simulink library "vehicleLE_cl"  (R2018b)
settings: Solver=VariableStepAuto  StartTime=0.0  StopTime=10.0  RelTol=1e-3
undefined symbols (not defined in the file): dragTurbine, dragTurbine_ul, env, fluidDynamicSurface, fluidDynamicSurface_cl, fuselage, fuselage_cl, surfaceCoefficients, surfaceCoefficients_ul, tethersMoment, tethersMoment_cl, thrAttachPtKinematics, thrAttachPtKinematics_ul, vhcl
libraries: vrlib x7, vectorNormalizer_ul x3, localApparentWind_ul x3, xProdMatrix_ul x2, dynamicPressure_ul x2, dspstat3 x2, dsppolyfun x2, firstOrderFilter_ul x1, simulink x1, alphaBetaLE_ul x1, rotateAboutVec x1, sixDoFDynamics_cl x1
settings Model: Creator=mcobb  LastModifiedBy=jldanie5

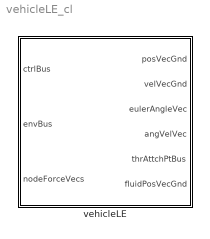
== system vehicleLE_cl ==
  vehicleLE : Subsystem  VariantControl=VSS_vehicle_vehicleLETest  mask{vcl=vhcl, rho=env.water.density.Value, grav=env.gravAccel.Value}
      mask prompts: vcl "Vehicle"; rho "Density"; grav "Gravity"
      mask DialogControl Container9 Prompt: General
      mask DialogControl Container5 Prompt: Vehicle object (OCT.vehicle)
      mask DialogControl ParameterGroupVar Prompt: Environment Object (OCT.env)
      mask Display:
      | image('kite.jpg',[100 100 601 528]/4,'on')
      | 
      | port_label('input',1,'ctrlBus')
      | port_label('input',2,'envBus')
      | port_label('input',3,'nodeForceVecs')
      | 
      | port_label('output',1,'posVecGnd')
      | port_label('output',2,'velVecGnd')
      | port_label('output',3,'eulAng')
      | port_label('output',4,'angVelVec')
      | port_label('output',5,'thrAttchPtBus')
      | port_label('output',6,'fluidPosVecGnd')

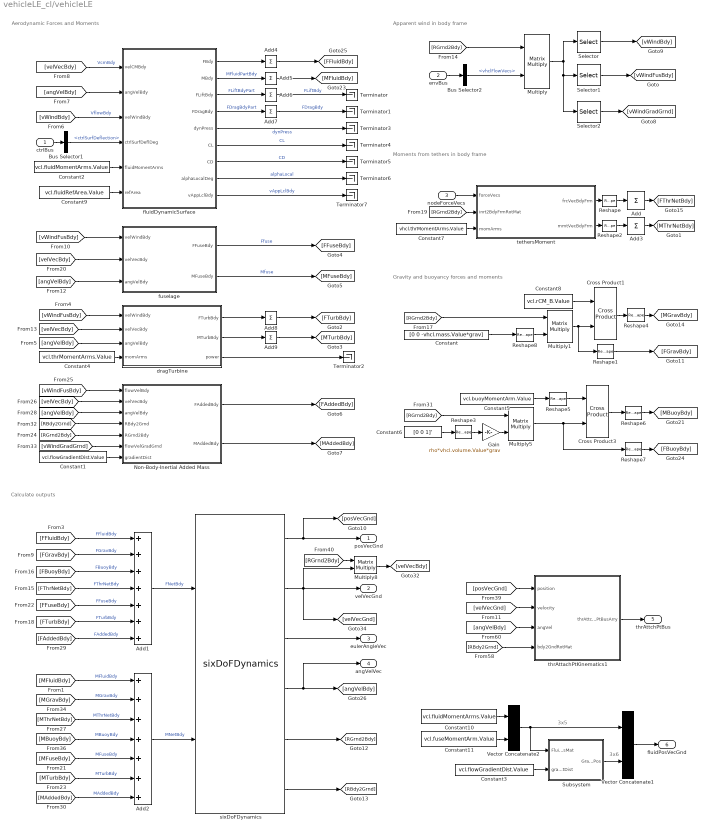
== system vehicleLE_cl/vehicleLE ==
  note: 3x6
  note: 3x5
  note: Calculate outputs
  note: Apparent wind in body frame
  note: Gravity and buoyancy forces and moments
  note: Moments from tethers in body frame
  note: Aerodynamic Forces and Moments
  ctrlBus : Inport  OutDataTypeStr=Bus: fltCtrlBus
  envBus : Inport  Port=2  OutDataTypeStr=Bus: envBus
  nodeForceVecs : Inport  Port=3
  Add : Sum  Inputs=+  CollapseMode=Specified dimension  CollapseDim=2
  Add1 : Sum  Inputs=+++++++
  Add2 : Sum  Inputs=+++++++
  Add3 : Sum  Inputs=+  CollapseMode=Specified dimension  CollapseDim=2
  Add{4..9} (6 alike) : Sum  Inputs=1  CollapseMode=Specified dimension  CollapseDim=2
  Bus Selector1 : BusSelector  OutputSignals=ctrlSurfDeflection
  Bus Selector2 : BusSelector  OutputSignals=vhclFlowVecs
  Constant : Constant  Value=[0 0 -vhcl.mass.Value*grav]
  Constant1 : Constant  Value=vcl.flowGradientDist.Value
  Constant10 : Constant  Value=vcl.fluidMomentArms.Value
  Constant11 : Constant  Value=vcl.fuseMomentArm.Value
  Constant2 : Constant  Value=vcl.fluidMomentArms.Value
  Constant3 : Constant  Value=vcl.flowGradientDist.Value
  Constant4 : Constant  Value=vcl.thrMomentArms.Value  VectorParams1D=off
  Constant5 : Constant  Value=vcl.buoyMomentArm.Value
  Constant6 : Constant  Value=[0 0 1]'
  Constant7 : Constant  Value=vhcl.thrMomentArms.Value
  Constant8 : Constant  Value=vcl.rCM_B.Value
  Constant9 : Constant  Value=vcl.fluidRefArea.Value
  Cross Product1 : vrlib/Utilities/Cross Product
      settings: SourceProductBaseCode=VR
  Cross Product3 : vrlib/Utilities/Cross Product
      settings: SourceProductBaseCode=VR
  Gain : Gain  Gain=rho*vhcl.volume.Value*grav
  Multiply{,1,5,8} (4 alike) : Product  Multiplication=Matrix(*)
  Non-Body-Inertial Added Mass : Subsystem  AncestorBlock=addedMass_cl/Non-Body-Inertial Added Mass  mask{MaMat=vcl.Ma6x6_B.Value}
      mask prompts: MaMat "Added Mass Matrix"
  Reshape : Reshape  OutputDimensionality=Customize  OutputDimensions=[3 vcl.numTethers.Value]
  Reshape{1,3..8} (7 alike) : Reshape  OutputDimensionality=Column vector (2-D)
  Reshape2 : Reshape  OutputDimensionality=Customize  OutputDimensions=[3 vcl.numTethers.Value]
  Selector : Selector  NumberOfDimensions=2  InputPortWidth=3  IndexOptions=Select all,Index vector (dialog)  Indices=[1 3],1:4  OutputSizes=1,1
  Selector1 : Selector  NumberOfDimensions=2  InputPortWidth=3  IndexOptions=Select all,Index vector (dialog)  Indices=[1 3],5  OutputSizes=1,1
  Selector2 : Selector  NumberOfDimensions=2  InputPortWidth=3  IndexOptions=Select all,Index vector (dialog)  Indices=[1 3],6:11  OutputSizes=1,1
  Subsystem : Subsystem
  Terminator{,1..7} (8 alike) : Terminator
  Vector Concatenate1 : Concatenate  Mode=Multidimensional array  ConcatenateDimension=2
  Vector Concatenate2 : Concatenate  Mode=Multidimensional array  ConcatenateDimension=2
  dragTurbine : Subsystem  AncestorBlock=dragTurbine_ul/dragTurbine  TreatAsAtomicUnit=on  mask{rho_fluid=rho, turb_struct=vcl.struct('OCT.turb'), momArms=0}
      mask prompts: rho_fluid "Fluid density"; turb_struct "Turbines structure"; momArms "Turbine Moment Arms"
  fluidDynamicSurface : Subsystem  AncestorBlock=fluidDynamicSurface_cl/fluidDynamicSurface  mask{aeroStruct=vcl.struct('OCT.aeroSurfLE'), fluidDensity=env.water.density.Value}
      mask prompts: aeroStruct "Aerodynamic surface structure"; fluidDensity "Fluid density"
      mask help:
      | Input must be an 1×N struct array with fields:
      |     refArea
      |     aeroCentPosVec
      |     spanUnitVec
      |     chordUnitVec
      |     CL
      |     CD
      |     alpha
      |     GainCL
      |     GainCD
      |
      | where N is the number of aerodynamic surfaces
      settings: MinAlgLoopOccurrences=on
  fuselage : Subsystem  AncestorBlock=fuselage_cl/fuselage  mask{momArm=vcl.fuseMomentArm.Value, fus=vcl.fuse, fusRhoDa=rho}
      mask prompts: momArm "Fuselage Moment Arm"; fus "Fuselage"; fusRhoDa "Density"
      mask DialogControl Container4 Prompt: General
      mask DialogControl Container9 Prompt: Fuselage object (OCT.fuselage)
      mask DialogControl Container8 Prompt: Environment Object (OCT.env)
  sixDoFDynamics : sixDoFDynamics_cl/sixDoFDynamics  vcl=vcl
  tethersMoment : Subsystem  AncestorBlock=tethersMoment_cl/tethersMoment  mask{arms=vcl.struct('OCT.thrAttchLE')}
      mask prompts: arms "Moment arm(s)"
  thrAttachPtKinematics1 : Subsystem  AncestorBlock=thrAttachPtKinematics_ul/thrAttachPtKinematics  InitFcn=thrAttachPtKinematics_init  mask{atchPts=vcl.struct('OCT.thrAttchLE')}
      mask prompts: atchPts "Tether attachment point vec in platform frame"
      mask init:
      | thrAttachPtKinematics_init
  posVecGnd : Outport
  velVecGnd : Outport  Port=2
  eulerAngleVec : Outport  Port=3
  angVelVec : Outport  Port=4
  thrAttchPtBus : Outport  Port=5
  fluidPosVecGnd : Outport  Port=6
  wires:
  sixDoFDynamics/3 -> eulerAngleVec/1
  sixDoFDynamics/1 -> [posVecGnd], posVecGnd/1
  sixDoFDynamics/2 -> Multiply8/2, [velVecGnd], velVecGnd/1
  thrAttachPtKinematics1/1(thrAttchPtBusArry) -> thrAttchPtBus/1
  fluidDynamicSurface/1(FBdy) -> Add4/1
  Constant2/1 -> fluidDynamicSurface/5(fluidMomentArms)
  fluidDynamicSurface/2(MBdy) -> Add5/1  "MFluidPartBdy"
  fluidDynamicSurface/3(FLiftBdy) -> Add6/1  "FLiftBdyPart"
  fluidDynamicSurface/4(FDragBdy) -> Add7/1  "FDragBdyPart"
  fluidDynamicSurface/5(dynPress) -> Terminator3/1  "dynPress"
  fluidDynamicSurface/6(CL) -> Terminator4/1  "CL"
  fluidDynamicSurface/7(CD) -> Terminator5/1  "CD"
  fluidDynamicSurface/8(alphaLocalDeg) -> Terminator6/1  "alphaLocal"
  fluidDynamicSurface/9(vAppLclBdy) -> Terminator7/1  "vAppLclBdy"
  Add4/1 -> [FFluidBdy]
  Add5/1 -> [MFluidBdy]
  Add6/1 -> Terminator/1  "FLiftBdy"
  Add7/1 -> Terminator1/1  "FDragBdy"
  [velVecBdy] -> fluidDynamicSurface/1(velCMBdy)  "VcmBdy"
  [angVelBdy] -> fluidDynamicSurface/2(angVelBdy)
  [vWindBdy] -> fluidDynamicSurface/3(velWindBdy)  "VflowBdy"
  Bus Selector1/1 -> fluidDynamicSurface/4(ctrlSurfDeflDeg)  "<ctrlSurfDeflection>"
  ctrlBus/1 -> Bus Selector1/1
  Constant9/1 -> fluidDynamicSurface/6(refArea)
  [vWindFusBdy] -> fuselage/1(velWindBdy)
  [velVecBdy] -> fuselage/2(velVecBdy)
  [angVelBdy] -> fuselage/3(angVelBdy)
  [vWindFusBdy] -> dragTurbine/1(velWindBdy)
  [velVecBdy] -> dragTurbine/2(velVecBdy)
  [angVelBdy] -> dragTurbine/3(angVelBdy)
  Constant4/1 -> dragTurbine/4(momArms)
  dragTurbine/1(FTurbBdy) -> Add8/1
  dragTurbine/2(MTurbBdy) -> Add9/1
  Add8/1 -> [FTurbBdy]
  Add9/1 -> [MTurbBdy]
  dragTurbine/3(power) -> Terminator2/1
  [vWindFusBdy] -> Non-Body-Inertial Added Mass/1("flowVelBdy ")
  [velVecBdy] -> Non-Body-Inertial Added Mass/2(velVecBdy)
  [angVelBdy] -> Non-Body-Inertial Added Mass/3(angVelBdy)
  [RBdy2Grnd] -> Non-Body-Inertial Added Mass/4(RBdy2Grnd)
  [RGrnd2Bdy] -> Non-Body-Inertial Added Mass/5(RGrnd2Bdy)
  [vWindGradGrnd] -> Non-Body-Inertial Added Mass/6(flowVelGradGrnd)
  Constant1/1 -> Non-Body-Inertial Added Mass/7(gradientDist)
  Non-Body-Inertial Added Mass/1(FAddedBdy) -> [FAddedBdy]
  Constant6/1 -> Reshape3/1
  Reshape3/1 -> Gain/1
  [RGrnd2Bdy] -> Multiply5/1
  Gain/1 -> Multiply5/2
  Constant5/1 -> Reshape5/1
  Reshape5/1 -> Cross Product3/1
  Cross Product3/1 -> Reshape6/1
  Reshape6/1 -> [MBuoyBdy]
  Multiply5/1 -> Reshape7/1, Cross Product3/2
  Reshape7/1 -> [FBuoyBdy]
  Reshape1/1 -> [FGravBdy]
  Multiply1/1 -> Reshape1/1, Cross Product1/2
  fuselage/1(FFuseBdy) -> [FFuseBdy]  "Ffuse"
  fuselage/2(MFuseBdy) -> [MFuseBdy]  "Mfuse"
  Constant/1 -> Reshape8/1
  [RGrnd2Bdy] -> Multiply1/1
  Reshape8/1 -> Multiply1/2
  Constant8/1 -> Cross Product1/1
  Cross Product1/1 -> Reshape4/1
  Reshape4/1 -> [MGravBdy]
  Constant7/1 -> tethersMoment/3(momArms)
  [RGrnd2Bdy] -> tethersMoment/2(inrt2BdyFrmRotMat)
  nodeForceVecs/1 -> tethersMoment/1(forceVecs)
  tethersMoment/1(frcVecBdyFrm) -> Reshape/1
  tethersMoment/2(mmtVecBdyFrm) -> Reshape2/1
  Reshape/1 -> Add/1
  Reshape2/1 -> Add3/1
  Add/1 -> [FThrNetBdy]
  Add3/1 -> [MThrNetBdy]
  [RGrnd2Bdy] -> Multiply/1
  envBus/1 -> Bus Selector2/1
  Bus Selector2/1 -> Multiply/2  "<vhclFlowVecs>"
  Multiply/1 -> Selector/1, Selector2/1, Selector1/1
  Selector/1 -> [vWindBdy]
  Selector1/1 -> [vWindFusBdy]
  Selector2/1 -> [vWindGradGrnd]
  [RGrnd2Bdy] -> Multiply8/1
  Multiply8/1 -> [velVecBdy]
  [FFluidBdy] -> Add1/1  "FFluidBdy"
  [FGravBdy] -> Add1/2  "FGravBdy"
  [FBuoyBdy] -> Add1/3  "FBuoyBdy"
  [FThrNetBdy] -> Add1/4  "FThrNetBdy"
  [FFuseBdy] -> Add1/5  "FFuseBdy"
  [FTurbBdy] -> Add1/6  "FTurbBdy"
  [FAddedBdy] -> Add1/7  "FAddedBdy"
  Add1/1 -> sixDoFDynamics/1  "FNetBdy"
  [MFluidBdy] -> Add2/1  "MFluidBdy"
  [MGravBdy] -> Add2/2  "MGravBdy"
  [MThrNetBdy] -> Add2/3  "MThrNetBdy"
  [MBuoyBdy] -> Add2/4  "MBuoyBdy"
  [MFuseBdy] -> Add2/5  "MFuseBdy"
  [MTurbBdy] -> Add2/6  "MTurbBdy"
  [MAddedBdy] -> Add2/7  "MAddedBdy"
  Add2/1 -> sixDoFDynamics/2  "MNetBdy"
  sixDoFDynamics/5 -> [RGrnd2Bdy]
  sixDoFDynamics/6 -> [RBdy2Grnd]
  [posVecGnd] -> thrAttachPtKinematics1/1(position)
  [velVecGnd] -> thrAttachPtKinematics1/2(velocity)
  [angVelBdy] -> thrAttachPtKinematics1/3(angVel)
  [RBdy2Grnd] -> thrAttachPtKinematics1/4(bdy2GndRotMat)
  Constant10/1 -> Vector Concatenate2/1
  Constant11/1 -> Vector Concatenate2/2
  Vector Concatenate2/1 -> Subsystem/1(FluidCentPosMat), Vector Concatenate1/1
  Constant3/1 -> Subsystem/2(gradientDist)
  Subsystem/1(GradientFlowPos) -> Vector Concatenate1/2
  Vector Concatenate1/1 -> fluidPosVecGnd/1
  sixDoFDynamics/4 -> [angVelBdy], angVelVec/1
  Non-Body-Inertial Added Mass/2(MAddedBdy) -> [MAddedBdy]

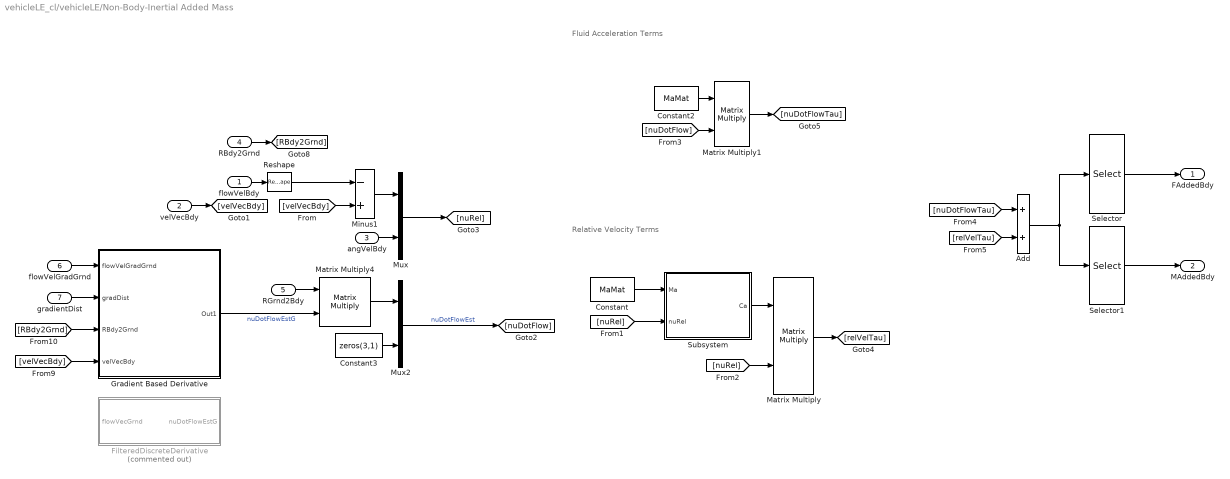
== system vehicleLE_cl/vehicleLE/Non-Body-Inertial Added Mass ==
  note: Relative Velocity Terms
  note: Fluid Acceleration Terms
  "flowVelBdy " : Inport
  velVecBdy : Inport  Port=2
  angVelBdy : Inport  Port=3
  RBdy2Grnd : Inport  Port=4
  RGrnd2Bdy : Inport  Port=5
  flowVelGradGrnd : Inport  Port=6
  gradientDist : Inport  Port=7
  Add : Sum
  Constant : Constant  Value=MaMat
  Constant2 : Constant  Value=MaMat
  Constant3 : Constant  Value=zeros(3,1)
  FilteredDiscreteDerivative : Subsystem  Commented=on
  Gradient Based Derivative : Subsystem
  Matrix Multiply : Product  Multiplication=Matrix(*)
  Matrix Multiply1 : Product  Multiplication=Matrix(*)
  Matrix Multiply4 : Product  Multiplication=Matrix(*)
  Minus1 : Sum  Inputs=-+
  Mux : Mux  Inputs=2
  Mux2 : Mux  Inputs=2
  Reshape : Reshape  OutputDimensionality=Column vector (2-D)
  Selector : Selector  InputPortWidth=6  IndexOptions=Index vector (dialog)  Indices=[1 2 3]  OutputSizes=1
  Selector1 : Selector  InputPortWidth=6  IndexOptions=Index vector (dialog)  Indices=[4 5 6]  OutputSizes=1
  Subsystem : Subsystem
  FAddedBdy : Outport
  MAddedBdy : Outport  Port=2
  wires:
  angVelBdy/1 -> Mux/2
  "flowVelBdy "/1 -> Reshape/1
  Constant/1 -> Subsystem/1(Ma)
  [nuRel] -> Subsystem/2(nuRel)
  Subsystem/1(Ca) -> Matrix Multiply/1
  [nuRel] -> Matrix Multiply/2
  Matrix Multiply/1 -> [relVelTau]
  Constant2/1 -> Matrix Multiply1/1
  [nuDotFlow] -> Matrix Multiply1/2
  Matrix Multiply1/1 -> [nuDotFlowTau]
  [relVelTau] -> Add/2
  [nuDotFlowTau] -> Add/1
  Add/1 -> Selector/1, Selector1/1
  Selector/1 -> FAddedBdy/1
  Selector1/1 -> MAddedBdy/1
  Constant3/1 -> Mux2/2
  Mux2/1 -> [nuDotFlow]  "nuDotFlowEst"
  RGrnd2Bdy/1 -> Matrix Multiply4/1
  Matrix Multiply4/1 -> Mux2/1
  Minus1/1 -> Mux/1
  Mux/1 -> [nuRel]
  velVecBdy/1 -> [velVecBdy]
  [velVecBdy] -> Minus1/2
  flowVelGradGrnd/1 -> Gradient Based Derivative/1(flowVelGradGrnd)
  gradientDist/1 -> Gradient Based Derivative/2(gradDist)
  [RBdy2Grnd] -> Gradient Based Derivative/3(RBdy2Grnd)
  [velVecBdy] -> Gradient Based Derivative/4(velVecBdy)
  RBdy2Grnd/1 -> [RBdy2Grnd]
  Gradient Based Derivative/1(Out1) -> Matrix Multiply4/2  "nuDotFlowEstG"
  Reshape/1 -> Minus1/1

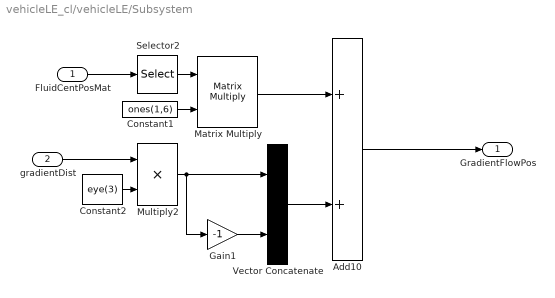
== system vehicleLE_cl/vehicleLE/Subsystem ==
  FluidCentPosMat : Inport
  gradientDist : Inport  Port=2
  Add10 : Sum
  Constant1 : Constant  Value=ones(1,6)  VectorParams1D=off
  Constant2 : Constant  Value=eye(3)
  Gain1 : Gain  Gain=-1
  Matrix Multiply : Product  Multiplication=Matrix(*)
  Multiply2 : Product
  Selector2 : Selector  NumberOfDimensions=2  InputPortWidth=3  IndexOptions=Select all,Index vector (dialog)  Indices=[1 3],5  OutputSizes=1,1
  Vector Concatenate : Concatenate  Mode=Multidimensional array  ConcatenateDimension=2
  GradientFlowPos : Outport
  wires:
  FluidCentPosMat/1 -> Selector2/1
  Vector Concatenate/1 -> Add10/2
  Selector2/1 -> Matrix Multiply/1
  Multiply2/1 -> Gain1/1, Vector Concatenate/1
  Constant1/1 -> Matrix Multiply/2
  Matrix Multiply/1 -> Add10/1
  Gain1/1 -> Vector Concatenate/2
  Constant2/1 -> Multiply2/2
  Add10/1 -> GradientFlowPos/1
  gradientDist/1 -> Multiply2/1

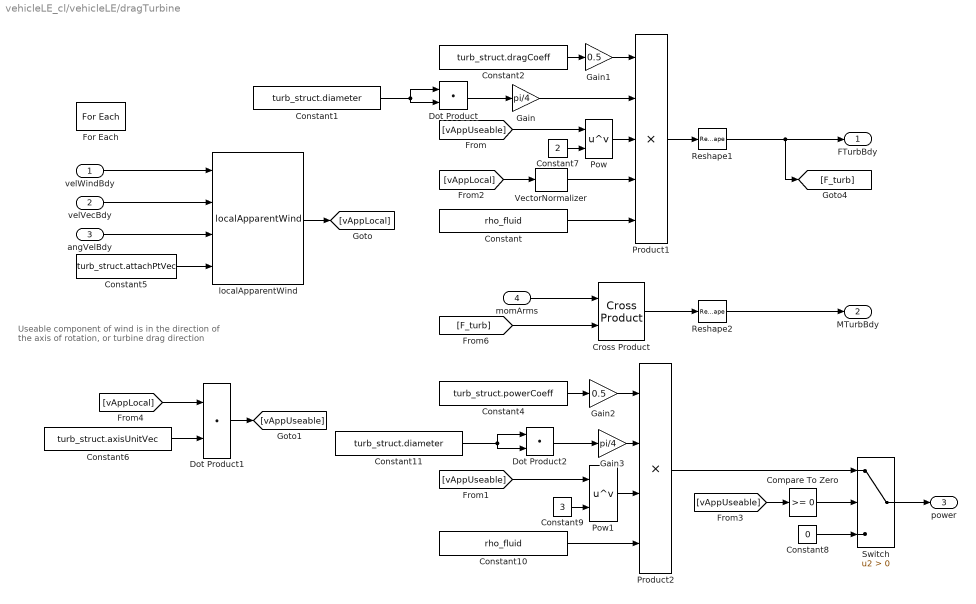
== system vehicleLE_cl/vehicleLE/dragTurbine ==
  note: Useable component of wind is in the direction of
      | the axis of rotation, or turbine drag direction
  velWindBdy : Inport
  velVecBdy : Inport  Port=2
  angVelBdy : Inport  Port=3
  momArms : Inport  Port=4
  Compare To Zero : simulink/Logic and Bit Operations/Compare To Zero  relop=>=  OutDataTypeStr=boolean
  Constant : Constant  Value=rho_fluid
  Constant1 : Constant  Value=turb_struct.diameter  VectorParams1D=off
  Constant10 : Constant  Value=rho_fluid
  Constant11 : Constant  Value=turb_struct.diameter  VectorParams1D=off
  Constant2 : Constant  Value=turb_struct.dragCoeff  VectorParams1D=off
  Constant4 : Constant  Value=turb_struct.powerCoeff  VectorParams1D=off
  Constant5 : Constant  Value=turb_struct.attachPtVec
  Constant6 : Constant  Value=turb_struct.axisUnitVec
  Constant7 : Constant  Value=2
  Constant8 : Constant  Value=0
  Constant9 : Constant  Value=3
  Cross Product : vrlib/Utilities/Cross Product
      settings: SourceProductBaseCode=VR
  Dot Product : DotProduct  InputSameDT=on  OutDataTypeStr=Inherit: Inherit via internal rule
  Dot Product1 : DotProduct  InputSameDT=on  OutDataTypeStr=Inherit: Inherit via internal rule
  Dot Product2 : DotProduct  InputSameDT=on  OutDataTypeStr=Inherit: Inherit via internal rule
  For Each : ForEach  DisableCoverage=on  IterateSubsysMaskParameter=off,on,off  SubsysMaskParameterIterationDimension=1,2,1  IndexMode=One-based
  Gain : Gain  Gain=pi/4
  Gain1 : Gain  Gain=0.5
  Gain2 : Gain  Gain=0.5
  Gain3 : Gain  Gain=pi/4
  Pow : Math  Operator=pow  RndMeth=Zero  SaturateOnIntegerOverflow=on
  Pow1 : Math  Operator=pow  RndMeth=Zero  SaturateOnIntegerOverflow=on
  Product1 : Product  Inputs=5
  Product2 : Product  Inputs=4
  Reshape1 : Reshape  OutputDimensionality=Column vector (2-D)
  Reshape2 : Reshape  OutputDimensionality=Column vector (2-D)
  Switch : Switch  Criteria=u2 > Threshold
  "VectorNormalizer " : vectorNormalizer_ul/VectorNormalizer   SystemSampleTime=-1
  localApparentWind : localApparentWind_ul/localApparentWind  SystemSampleTime=-1
  FTurbBdy : Outport  PortDimensions=[3,1]  ConcatenationDimension=2
  MTurbBdy : Outport  Port=2  PortDimensions=[3,1]  ConcatenationDimension=2
  power : Outport  Port=3  PortDimensions=[1,1]  ConcatenationDimension=2
  wires:
  Cross Product/1 -> Reshape2/1
  Product1/1 -> Reshape1/1
  Product2/1 -> Switch/1
  Constant2/1 -> Gain1/1
  momArms/1 -> Cross Product/1
  [F_turb] -> Cross Product/2
  Reshape1/1 -> FTurbBdy/1, [F_turb]
  Reshape2/1 -> MTurbBdy/1
  velVecBdy/1 -> localApparentWind/2
  angVelBdy/1 -> localApparentWind/3
  velWindBdy/1 -> localApparentWind/1
  localApparentWind/1 -> [vAppLocal]
  Constant5/1 -> localApparentWind/4
  Constant6/1 -> Dot Product1/2
  [vAppUseable] -> Pow/1
  "VectorNormalizer "/1 -> Product1/4
  Constant1/1 -> Dot Product/1, Dot Product/2
  Constant9/1 -> Pow1/2
  Dot Product1/1 -> [vAppUseable]
  Gain1/1 -> Product1/1
  Constant/1 -> Product1/5
  Constant10/1 -> Product2/4
  Gain2/1 -> Product2/1
  Constant4/1 -> Gain2/1
  Pow1/1 -> Product2/3
  Pow/1 -> Product1/3
  Constant7/1 -> Pow/2
  [vAppLocal] -> "VectorNormalizer "/1
  Switch/1 -> power/1
  Compare To Zero/1 -> Switch/2
  [vAppUseable] -> Compare To Zero/1
  Constant8/1 -> Switch/3
  [vAppLocal] -> Dot Product1/1
  [vAppUseable] -> Pow1/1
  Dot Product/1 -> Gain/1
  Gain/1 -> Product1/2
  Dot Product2/1 -> Gain3/1
  Constant11/1 -> Dot Product2/2, Dot Product2/1
  Gain3/1 -> Product2/2

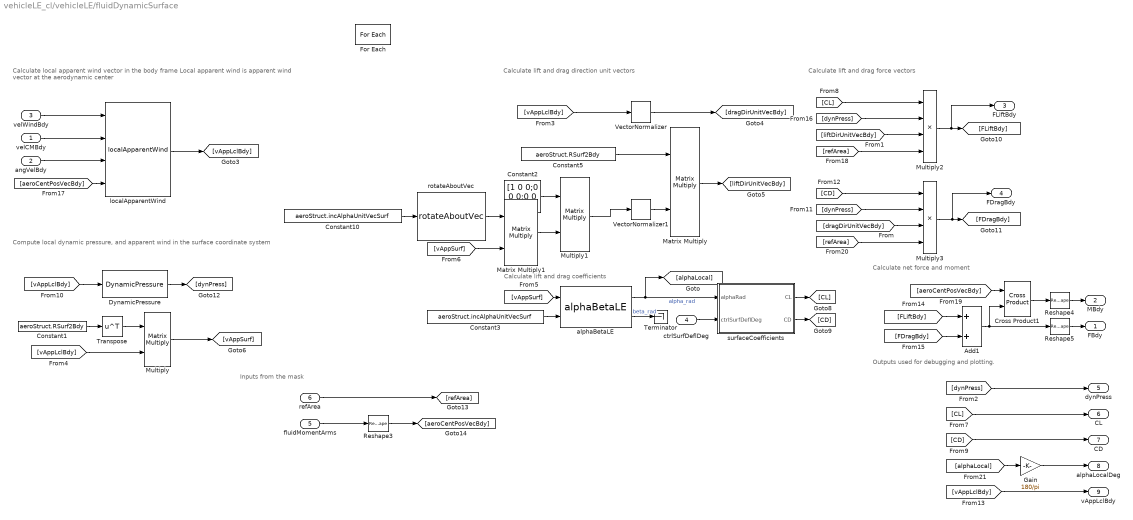
== system vehicleLE_cl/vehicleLE/fluidDynamicSurface ==
  note: Outputs used for debugging and plotting.
  note: Calculate net force and moment
  note: Calculate lift and drag force vectors
  note: Calculate lift and drag coefficients
  note: Compute local dynamic pressure,
      | and apparent wind in the surface coordinate system
  note: Inputs from the mask
  note: Calculate lift and drag direction unit vectors
  note: Calculate local apparent wind vector in the body frame
      | Local apparent wind is apparent wind vector at the aerodynamic center
  velCMBdy : Inport
  angVelBdy : Inport  Port=2
  velWindBdy : Inport  Port=3  Partition=on  PartitionDimension=2  PartitionWidth=1  PartitionOffset=0
  ctrlSurfDeflDeg : Inport  Port=4  Partition=on  PartitionDimension=1  PartitionWidth=1  PartitionOffset=0
  fluidMomentArms : Inport  Port=5  Partition=on  PartitionDimension=2  PartitionWidth=1  PartitionOffset=0
  refArea : Inport  Port=6
  Add1 : Sum
  Constant1 : Constant  Value=aeroStruct.RSurf2Bdy
  Constant10 : Constant  Value=aeroStruct.incAlphaUnitVecSurf
  Constant2 : Constant  Value=[1 0 0;0 0 0;0 0 1]
  Constant3 : Constant  Value=aeroStruct.incAlphaUnitVecSurf
  Constant5 : Constant  Value=aeroStruct.RSurf2Bdy
  Cross Product1 : vrlib/Utilities/Cross Product
      settings: SourceProductBaseCode=VR
  DynamicPressure : dynamicPressure_ul/DynamicPressure  rho=fluidDensity
  For Each : ForEach  DisableCoverage=on  IterateSubsysMaskParameter=on,off  SubsysMaskParameterIterationDimension=2,1  IndexMode=One-based
  Gain : Gain  Gain=180/pi
  Matrix Multiply : Product  Multiplication=Matrix(*)
  Matrix Multiply1 : Product  Multiplication=Matrix(*)
  Multiply : Product  Multiplication=Matrix(*)
  Multiply1 : Product  Multiplication=Matrix(*)
  Multiply2 : Product  Inputs=4
  Multiply3 : Product  Inputs=4
  Reshape3 : Reshape  OutputDimensionality=Column vector (2-D)
  Reshape4 : Reshape  OutputDimensionality=Column vector (2-D)
  Reshape5 : Reshape  OutputDimensionality=Column vector (2-D)
  Terminator : Terminator
  Transpose : Math  Operator=transpose  SaturateOnIntegerOverflow=on
  "VectorNormalizer " : vectorNormalizer_ul/VectorNormalizer   SystemSampleTime=-1
  VectorNormalizer1 : vectorNormalizer_ul/VectorNormalizer   SystemSampleTime=-1
  alphaBetaLE : alphaBetaLE_ul/alphaBetaLE  SystemSampleTime=-1
  localApparentWind : localApparentWind_ul/localApparentWind  SystemSampleTime=-1
  rotateAboutVec : rotateAboutVec/rotateAboutVec  ang=90
  surfaceCoefficients : Subsystem  AncestorBlock=surfaceCoefficients_ul/surfaceCoefficients
  FBdy : Outport  ConcatenationDimension=2
  MBdy : Outport  Port=2  PortDimensions=[3 1]  ConcatenationDimension=2
  FLiftBdy : Outport  Port=3  ConcatenationDimension=2
  FDragBdy : Outport  Port=4  ConcatenationDimension=2
  dynPress : Outport  Port=5  ConcatenationDimension=2
  CL : Outport  Port=6  ConcatenationDimension=2
  CD : Outport  Port=7  ConcatenationDimension=2
  alphaLocalDeg : Outport  Port=8  ConcatenationDimension=2
  vAppLclBdy : Outport  Port=9  ConcatenationDimension=2
  wires:
  Constant3/1 -> alphaBetaLE/2
  Constant10/1 -> rotateAboutVec/1
  Multiply1/1 -> VectorNormalizer1/1
  Matrix Multiply1/1 -> Multiply1/2
  Constant2/1 -> Multiply1/1
  rotateAboutVec/1 -> Matrix Multiply1/1
  [vAppSurf] -> Matrix Multiply1/2
  Transpose/1 -> Multiply/1
  velWindBdy/1 -> localApparentWind/1
  [vAppLclBdy] -> "VectorNormalizer "/1
  "VectorNormalizer "/1 -> [dragDirUnitVecBdy]
  Constant1/1 -> Transpose/1
  [vAppLclBdy] -> Multiply/2
  Multiply/1 -> [vAppSurf]
  [vAppSurf] -> alphaBetaLE/1
  alphaBetaLE/2 -> Terminator/1  "beta_rad"
  surfaceCoefficients/1(CL) -> [CL]
  surfaceCoefficients/2(CD) -> [CD]
  [CL] -> Multiply2/1
  DynamicPressure/1 -> [dynPress]
  [liftDirUnitVecBdy] -> Multiply2/3
  [vAppLclBdy] -> DynamicPressure/1
  Multiply2/1 -> FLiftBdy/1, [FLiftBdy]
  Multiply3/1 -> FDragBdy/1, [FDragBdy]
  [dragDirUnitVecBdy] -> Multiply3/3
  [dynPress] -> Multiply3/2
  [CD] -> Multiply3/1
  Add1/1 -> Reshape5/1, Cross Product1/2
  [FDragBdy] -> Add1/2
  [FLiftBdy] -> Add1/1
  Matrix Multiply/1 -> [liftDirUnitVecBdy]
  Constant5/1 -> Matrix Multiply/1
  VectorNormalizer1/1 -> Matrix Multiply/2
  [dynPress] -> Multiply2/2
  Cross Product1/1 -> Reshape4/1
  fluidMomentArms/1 -> Reshape3/1
  [refArea] -> Multiply2/4
  [refArea] -> Multiply3/4
  [aeroCentPosVecBdy] -> Cross Product1/1
  refArea/1 -> [refArea]
  Reshape3/1 -> [aeroCentPosVecBdy]
  Reshape4/1 -> MBdy/1
  Reshape5/1 -> FBdy/1
  ctrlSurfDeflDeg/1 -> surfaceCoefficients/2(ctrlSurfDeflDeg)
  alphaBetaLE/1 -> surfaceCoefficients/1(alphaRad), [alphaLocal]  "alpha_rad"
  velCMBdy/1 -> localApparentWind/2
  angVelBdy/1 -> localApparentWind/3
  [aeroCentPosVecBdy] -> localApparentWind/4
  localApparentWind/1 -> [vAppLclBdy]
  [dynPress] -> dynPress/1
  [CD] -> CD/1
  [CL] -> CL/1
  Gain/1 -> alphaLocalDeg/1
  [vAppLclBdy] -> vAppLclBdy/1
  [alphaLocal] -> Gain/1

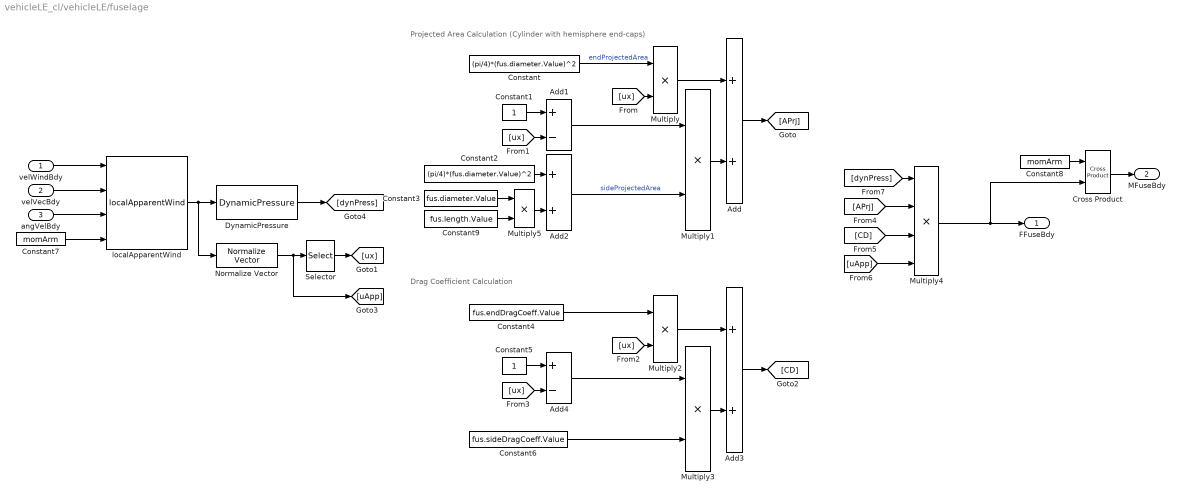
== system vehicleLE_cl/vehicleLE/fuselage ==
  note: Drag Coefficient Calculation
  note: Projected Area Calculation (Cylinder with hemisphere end-caps)
  velWindBdy : Inport
  velVecBdy : Inport  Port=2
  angVelBdy : Inport  Port=3
  Add : Sum
  Add1 : Sum  Inputs=+-
  Add2 : Sum
  Add3 : Sum
  Add4 : Sum  Inputs=+-
  Constant : Constant  Value=(pi/4)*(fus.diameter.Value)^2
  Constant1 : Constant
  Constant2 : Constant  Value=(pi/4)*(fus.diameter.Value)^2
  Constant3 : Constant  Value=fus.diameter.Value
  Constant4 : Constant  Value=fus.endDragCoeff.Value
  Constant5 : Constant
  Constant6 : Constant  Value=fus.sideDragCoeff.Value
  Constant7 : Constant  Value=momArm
  Constant8 : Constant  Value=momArm
  Constant9 : Constant  Value=fus.length.Value
  Cross Product : vrlib/Utilities/Cross Product
      settings: SourceProductBaseCode=VR
  DynamicPressure : dynamicPressure_ul/DynamicPressure  rho=fusRhoDa
  Multiply{,1..3,5} (5 alike) : Product
  Multiply4 : Product  Inputs=4
  Normalize Vector : vrlib/Utilities/Normalize Vector  maxzero=0
      settings: SourceProductName=Simulink 3D Animation  SourceProductBaseCode=VR
  Selector : Selector  InputPortWidth=3  IndexOptions=Index vector (dialog)  Indices=1  OutputSizes=1
  localApparentWind : localApparentWind_ul/localApparentWind  SystemSampleTime=-1
  FFuseBdy : Outport
  MFuseBdy : Outport  Port=2
  wires:
  Normalize Vector/1 -> [uApp], Selector/1
  Add/1 -> [APrj]
  Selector/1 -> [ux]
  Multiply1/1 -> Add/2
  Multiply/1 -> Add/1
  Constant/1 -> Multiply/1  "endProjectedArea"
  [ux] -> Multiply/2
  Add1/1 -> Multiply1/1
  Constant1/1 -> Add1/1
  [ux] -> Add1/2
  Add2/1 -> Multiply1/2  "sideProjectedArea"
  Constant2/1 -> Add2/1
  [ux] -> Add4/2
  Constant5/1 -> Add4/1
  Add4/1 -> Multiply3/1
  [ux] -> Multiply2/2
  Multiply2/1 -> Add3/1
  Multiply3/1 -> Add3/2
  Constant6/1 -> Multiply3/2
  Constant4/1 -> Multiply2/1
  Add3/1 -> [CD]
  Multiply4/1 -> Cross Product/2, FFuseBdy/1
  [dynPress] -> Multiply4/1
  [APrj] -> Multiply4/2
  [CD] -> Multiply4/3
  [uApp] -> Multiply4/4
  angVelBdy/1 -> localApparentWind/3
  localApparentWind/1 -> Normalize Vector/1, DynamicPressure/1
  velVecBdy/1 -> localApparentWind/2
  Constant7/1 -> localApparentWind/4
  velWindBdy/1 -> localApparentWind/1
  DynamicPressure/1 -> [dynPress]
  Constant8/1 -> Cross Product/1
  Cross Product/1 -> MFuseBdy/1
  Multiply5/1 -> Add2/2
  Constant3/1 -> Multiply5/1
  Constant9/1 -> Multiply5/2

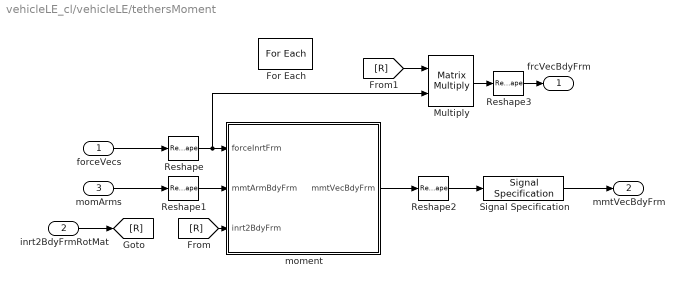
== system vehicleLE_cl/vehicleLE/tethersMoment ==
  forceVecs : Inport  Partition=on  PartitionDimension=3  PartitionWidth=1  PartitionOffset=0
  inrt2BdyFrmRotMat : Inport  Port=2
  momArms : Inport  Port=3  Partition=on  PartitionDimension=2  PartitionWidth=1  PartitionOffset=0
  For Each : ForEach  DisableCoverage=on  IterateSubsysMaskParameter=on  SubsysMaskParameterIterationDimension=2  IndexMode=One-based
  Multiply : Product  Multiplication=Matrix(*)
  Reshape{,1..3} (4 alike) : Reshape  OutputDimensionality=Column vector (2-D)
  Signal Specification : SignalSpecification  Dimensions=[3 1]
  moment : Subsystem
  frcVecBdyFrm : Outport  ConcatenationDimension=2
  mmtVecBdyFrm : Outport  Port=2  ConcatenationDimension=2
  wires:
  Reshape/1 -> Multiply/2, moment/1(forceInrtFrm)
  moment/1(mmtVecBdyFrm) -> Reshape2/1
  inrt2BdyFrmRotMat/1 -> [R]
  momArms/1 -> Reshape1/1
  forceVecs/1 -> Reshape/1
  [R] -> moment/3(inrt2BdyFrm)
  Multiply/1 -> Reshape3/1
  [R] -> Multiply/1
  Reshape1/1 -> moment/2(mmtArmBdyFrm)
  Reshape2/1 -> Signal Specification/1
  Reshape3/1 -> frcVecBdyFrm/1
  Signal Specification/1 -> mmtVecBdyFrm/1

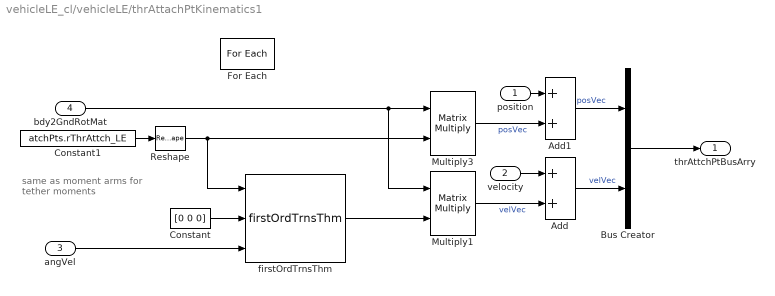
== system vehicleLE_cl/vehicleLE/thrAttachPtKinematics1 ==
  note: same as moment arms
      | for tether moments
  position : Inport
  velocity : Inport  Port=2
  angVel : Inport  Port=3
  bdy2GndRotMat : Inport  Port=4
  Add : Sum
  Add1 : Sum
  Bus Creator : BusCreator  Inputs=2  OutDataTypeStr=Bus: thrAttachPtKinematicsBus  NonVirtualBus=on
  Constant : Constant  Value=[0 0 0]
  Constant1 : Constant  Value=atchPts.rThrAttch_LE
  For Each : ForEach  DisableCoverage=on  IterateSubsysMaskParameter=on  SubsysMaskParameterIterationDimension=2  IndexMode=One-based
  Multiply1 : Product  Multiplication=Matrix(*)
  Multiply3 : Product  Multiplication=Matrix(*)
  Reshape : Reshape  OutputDimensionality=Column vector (2-D)
  firstOrdTrnsThm : firstOrdTrnsThm_ul/firstOrdTrnsThm  SystemSampleTime=-1
  thrAttchPtBusArry : Outport  ConcatenationDimension=1
  wires:
  Reshape/1 -> firstOrdTrnsThm/1, Multiply3/2
  Multiply3/1 -> Add1/2  "posVec"
  Multiply1/1 -> Add/2  "velVec"
  velocity/1 -> Add/1
  position/1 -> Add1/1
  Bus Creator/1 -> thrAttchPtBusArry/1
  Constant1/1 -> Reshape/1
  angVel/1 -> firstOrdTrnsThm/3
  firstOrdTrnsThm/1 -> Multiply1/2
  Constant/1 -> firstOrdTrnsThm/2
  bdy2GndRotMat/1 -> Multiply1/1, Multiply3/1
  Add/1 -> Bus Creator/2  "velVec"
  Add1/1 -> Bus Creator/1  "posVec"

== system vehicleLE_cl/vehicleLE/Non-Body-Inertial Added Mass/FilteredDiscreteDerivative ==
  flowVecGrnd : Inport
  Clock : Clock
  Divide : Product  Inputs=*/
  Memory : Memory
  Memory1 : Memory  InitialCondition=-.01
  Minus : Sum  Inputs=+-
  Minus2 : Sum  Inputs=+-
  firstOrderFilter : firstOrderFilter_ul/firstOrderFilter  tau=.01  ic=zeros(3,1)
  nuDotFlowEstG : Outport
  wires:
  Divide/1 -> firstOrderFilter/1
  flowVecGrnd/1 -> Minus/1, Memory/1
  Minus2/1 -> Divide/2  "samp"
  Clock/1 -> Minus2/1, Memory1/1
  Memory1/1 -> Minus2/2
  Minus/1 -> Divide/1
  Memory/1 -> Minus/2
  firstOrderFilter/1 -> nuDotFlowEstG/1  "nuDotFlowEstG"

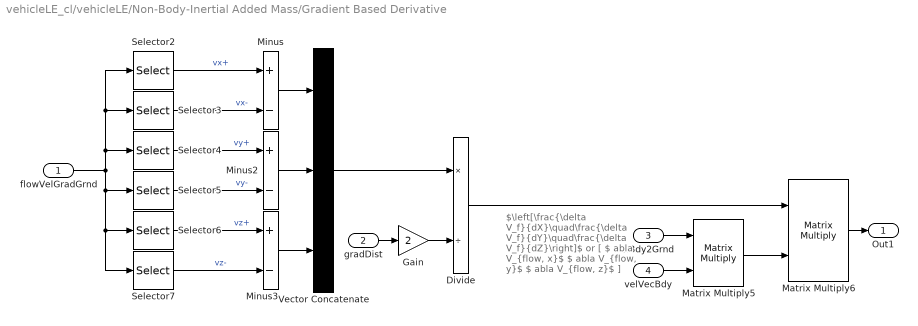
== system vehicleLE_cl/vehicleLE/Non-Body-Inertial Added Mass/Gradient Based Derivative ==
  note: $\left[\frac{\delta V_f}{dX}\quad\frac{\delta V_f}{dY}\quad\frac{\delta V_f}{dZ}\right]$
      | or
      | [ $\nabla V_{flow, x}$
      | $\nabla V_{flow, y}$
      | $\nabla V_{flow, z}$ ]
  flowVelGradGrnd : Inport
  gradDist : Inport  Port=2
  RBdy2Grnd : Inport  Port=3
  velVecBdy : Inport  Port=4
  Divide : Product  Inputs=*/
  Gain : Gain  Gain=2
  Matrix Multiply5 : Product  Multiplication=Matrix(*)
  Matrix Multiply6 : Product  Multiplication=Matrix(*)
  Minus : Sum  Inputs=+-
  Minus2 : Sum  Inputs=+-
  Minus3 : Sum  Inputs=+-
  Selector2 : Selector  NumberOfDimensions=2  InputPortWidth=3  IndexOptions=Select all,Index vector (dialog)  Indices=[1 3],1  OutputSizes=1,1
  Selector3 : Selector  NumberOfDimensions=2  InputPortWidth=3  IndexOptions=Select all,Index vector (dialog)  Indices=[1 3],4  OutputSizes=1,1
  Selector4 : Selector  NumberOfDimensions=2  InputPortWidth=3  IndexOptions=Select all,Index vector (dialog)  Indices=[1 3],2  OutputSizes=1,1
  Selector5 : Selector  NumberOfDimensions=2  InputPortWidth=3  IndexOptions=Select all,Index vector (dialog)  Indices=[1 3],5  OutputSizes=1,1
  Selector6 : Selector  NumberOfDimensions=2  InputPortWidth=3  IndexOptions=Select all,Index vector (dialog)  Indices=[1 3],3  OutputSizes=1,1
  Selector7 : Selector  NumberOfDimensions=2  InputPortWidth=3  IndexOptions=Select all,Index vector (dialog)  Indices=[1 3],1  OutputSizes=1,1
  Vector Concatenate : Concatenate  NumInputs=3  Mode=Multidimensional array  ConcatenateDimension=2
  Out1 : Outport
  wires:
  velVecBdy/1 -> Matrix Multiply5/2
  Minus/1 -> Vector Concatenate/1
  Matrix Multiply5/1 -> Matrix Multiply6/2
  Selector7/1 -> Minus3/2  "vz-"
  Minus2/1 -> Vector Concatenate/2
  Vector Concatenate/1 -> Divide/1
  Selector6/1 -> Minus3/1  "vz+"
  Selector4/1 -> Minus2/1  "vy+"
  gradDist/1 -> Gain/1
  Selector5/1 -> Minus2/2  "vy-"
  flowVelGradGrnd/1 -> Selector4/1, Selector3/1, Selector2/1, Selector5/1, Selector6/1, Selector7/1
  Minus3/1 -> Vector Concatenate/3
  Gain/1 -> Divide/2
  RBdy2Grnd/1 -> Matrix Multiply5/1
  Selector3/1 -> Minus/2  "vx-"
  Selector2/1 -> Minus/1  "vx+"
  Divide/1 -> Matrix Multiply6/1
  Matrix Multiply6/1 -> Out1/1

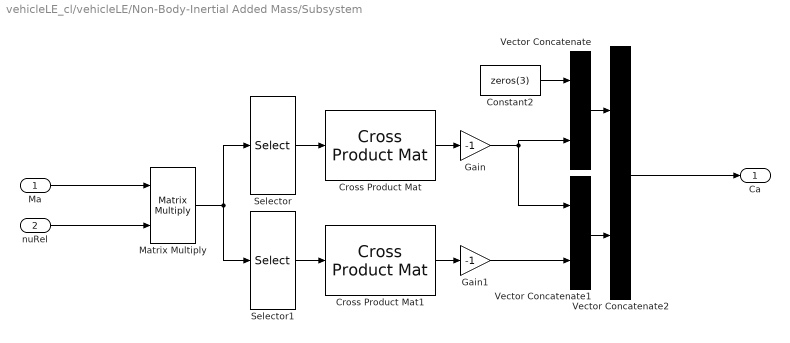
== system vehicleLE_cl/vehicleLE/Non-Body-Inertial Added Mass/Subsystem ==
  Ma : Inport
  nuRel : Inport  Port=2
  Constant2 : Constant  Value=zeros(3)
  Cross Product Mat : xProdMatrix_ul/Cross Product Mat  SystemSampleTime=-1
  Cross Product Mat1 : xProdMatrix_ul/Cross Product Mat  SystemSampleTime=-1
  Gain : Gain  Gain=-1
  Gain1 : Gain  Gain=-1
  Matrix Multiply : Product  Multiplication=Matrix(*)
  Selector : Selector  InputPortWidth=6  IndexOptions=Index vector (dialog)  Indices=[1 2 3]  OutputSizes=1
  Selector1 : Selector  InputPortWidth=6  IndexOptions=Index vector (dialog)  Indices=[4 5 6]  OutputSizes=1
  Vector Concatenate : Concatenate  Mode=Multidimensional array  ConcatenateDimension=2
  Vector Concatenate1 : Concatenate  Mode=Multidimensional array  ConcatenateDimension=2
  Vector Concatenate2 : Concatenate  Mode=Multidimensional array
  Ca : Outport
  wires:
  Gain/1 -> Vector Concatenate1/1, Vector Concatenate/2
  Ma/1 -> Matrix Multiply/1
  Selector/1 -> Cross Product Mat/1
  Matrix Multiply/1 -> Selector/1, Selector1/1
  Selector1/1 -> Cross Product Mat1/1
  Cross Product Mat1/1 -> Gain1/1
  Vector Concatenate1/1 -> Vector Concatenate2/2
  Cross Product Mat/1 -> Gain/1
  Gain1/1 -> Vector Concatenate1/2
  Vector Concatenate/1 -> Vector Concatenate2/1
  Constant2/1 -> Vector Concatenate/1
  nuRel/1 -> Matrix Multiply/2
  Vector Concatenate2/1 -> Ca/1

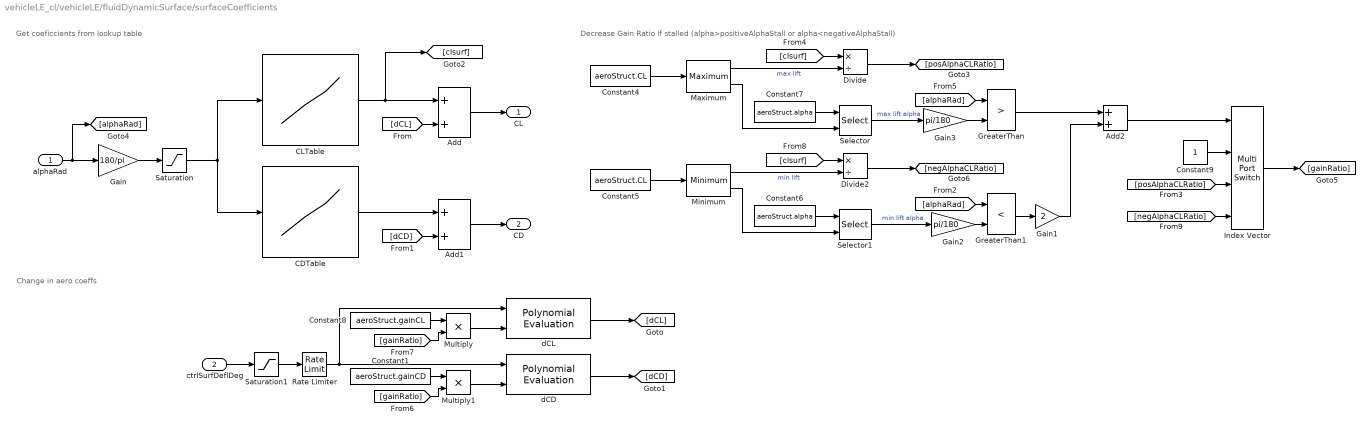
== system vehicleLE_cl/vehicleLE/fluidDynamicSurface/surfaceCoefficients ==
  note: Change in aero coeffs
  note: Decrease Gain Ratio if stalled (alpha>positiveAlphaStall or alpha<negativeAlphaStall)
  note: Get coeficcients from lookup table
  alphaRad : Inport
  ctrlSurfDeflDeg : Inport  Port=2
  Add : Sum
  Add1 : Sum
  Add2 : Sum
  CDTable : Lookup_n-D  NumberOfTableDimensions=1  LookupTableObject=CLTable  BreakpointsForDimension1=aeroStruct.alpha  Table=aeroStruct.CD  ExtrapMethod=Clip  UseLastTableValue=on  InternalRulePriority=Speed  RndMeth=Simplest  InputSameDT=on
  CLTable : Lookup_n-D  NumberOfTableDimensions=1  LookupTableObject=CLTable  BreakpointsForDimension1=aeroStruct.alpha  Table=aeroStruct.CL  ExtrapMethod=Clip  UseLastTableValue=on  InternalRulePriority=Speed  RndMeth=Simplest  InputSameDT=on
  Constant1 : Constant  Value=aeroStruct.gainCD
  Constant4 : Constant  Value=aeroStruct.CL
  Constant5 : Constant  Value=aeroStruct.CL
  Constant6 : Constant  Value=aeroStruct.alpha
  Constant7 : Constant  Value=aeroStruct.alpha
  Constant8 : Constant  Value=aeroStruct.gainCL
  Constant9 : Constant
  Divide : Product  Inputs=*/
  Divide2 : Product  Inputs=*/
  Gain : Gain  Gain=180/pi
  Gain1 : Gain  Gain=2
  Gain2 : Gain  Gain=pi/180
  Gain3 : Gain  Gain=pi/180
  GreaterThan : RelationalOperator  Operator=>  OutDataTypeStr=boolean  RndMeth=Simplest
  GreaterThan1 : RelationalOperator  Operator=<  OutDataTypeStr=boolean  RndMeth=Simplest
  Index Vector : MultiPortSwitch  DataPortOrder=Zero-based contiguous  zeroidx=on
  Maximum : dspstat3/Maximum  operation=maximum  fcn=Value and Index  indexBase=One  operateOver=Each column  Dimension=1  InputProcessing=Columns as channels (frame based)  reset=None  roiEnable=off  roiType=Rectangles  roiPortion=Entire ROI  roiOutput=Individual statistics for each ROI  roiFlag=off  roundingMode=Floor  overflowMode=off  accumDataTypeStr=Inherit: Same as product output  accumLastDataTypeStr=Inherit: Same as product output
  Minimum : dspstat3/Minimum  operation=minimum  fcn=Value and Index  indexBase=One  operateOver=Each column  Dimension=1  InputProcessing=Columns as channels (frame based)  reset=None  roiEnable=off  roiType=Rectangles  roiPortion=Entire ROI  roiOutput=Individual statistics for each ROI  roiFlag=off  roundingMode=Floor  overflowMode=off
      settings: SourceProductName=DSP System Toolbox  SourceProductBaseCode=DS
  Multiply : Product
  Multiply1 : Product
  Rate Limiter : RateLimiter  RisingSlewLimit=aeroStruct.maxCtrlDefSpeed  FallingSlewLimit=-aeroStruct.maxCtrlDefSpeed  SampleTimeMode=inherited
  Saturation : Saturate  UpperLimit=90  LowerLimit=-90
  Saturation1 : Saturate  UpperLimit=aeroStruct.maxCtrlDef  LowerLimit=aeroStruct.minCtrlDef
  Selector : Selector  InputPortWidth=length(vhcl.portWing.alpha.Value)  IndexOptions=Index vector (port)  Indices=[1 3]  OutputSizes=1
  Selector1 : Selector  InputPortWidth=length(vhcl.portWing.alpha.Value)  IndexOptions=Index vector (port)  Indices=[1 3]  OutputSizes=1
  dCD : dsppolyfun/Polynomial Evaluation  useConstCoeffs=off  constCoeffs=[0]
      settings: SourceProductName=DSP System Toolbox  SourceProductBaseCode=DS
  dCL : dsppolyfun/Polynomial Evaluation  useConstCoeffs=off  constCoeffs=[0]
      settings: SourceProductName=DSP System Toolbox  SourceProductBaseCode=DS
  CL : Outport
  CD : Outport  Port=2
  wires:
  Saturation1/1 -> Rate Limiter/1
  Gain3/1 -> GreaterThan/2
  Gain2/1 -> GreaterThan1/2
  Constant1/1 -> Multiply1/1
  [gainRatio] -> Multiply1/2
  Multiply/1 -> dCL/2
  [gainRatio] -> Multiply/2
  Constant8/1 -> Multiply/1
  Index Vector/1 -> [gainRatio]
  [posAlphaCLRatio] -> Index Vector/3
  [negAlphaCLRatio] -> Index Vector/4
  Constant9/1 -> Index Vector/2
  Add2/1 -> Index Vector/1
  Gain1/1 -> Add2/2
  GreaterThan/1 -> Add2/1
  GreaterThan1/1 -> Gain1/1
  [alphaRad] -> GreaterThan1/1
  Selector1/1 -> Gain2/1  "min lift alpha"
  Constant5/1 -> Minimum/1
  Constant6/1 -> Selector1/1
  Minimum/1 -> Divide2/2  "min lift"
  Divide2/1 -> [negAlphaCLRatio]
  [clsurf] -> Divide2/1
  Minimum/2 -> Selector1/2
  [alphaRad] -> GreaterThan/1
  [clsurf] -> Divide/1
  Maximum/1 -> Divide/2  "max lift"
  Divide/1 -> [posAlphaCLRatio]
  Selector/1 -> Gain3/1  "max lift alpha"
  Maximum/2 -> Selector/2
  Constant7/1 -> Selector/1
  alphaRad/1 -> Gain/1, [alphaRad]
  Constant4/1 -> Maximum/1
  Saturation/1 -> CDTable/1, CLTable/1
  ctrlSurfDeflDeg/1 -> Saturation1/1
  Rate Limiter/1 -> dCD/1, dCL/1
  Multiply1/1 -> dCD/2
  CDTable/1 -> Add1/1
  [dCD] -> Add1/2
  Add1/1 -> CD/1
  Add/1 -> CL/1
  CLTable/1 -> Add/1, [clsurf]
  [dCL] -> Add/2
  dCD/1 -> [dCD]
  dCL/1 -> [dCL]
  Gain/1 -> Saturation/1

== system vehicleLE_cl/vehicleLE/tethersMoment/moment ==
  forceInrtFrm : Inport
  mmtArmBdyFrm : Inport  Port=2
  inrt2BdyFrm : Inport  Port=3
  Cross Product : vrlib/Utilities/Cross Product
      settings: SourceProductBaseCode=VR
  Multiply : Product  Multiplication=Matrix(*)
  Reshape : Reshape  OutputDimensionality=Column vector (2-D)
  Reshape1 : Reshape  OutputDimensionality=Column vector (2-D)
  mmtVecBdyFrm : Outport
  wires:
  Reshape1/1 -> Cross Product/1
  Reshape/1 -> Multiply/2
  Cross Product/1 -> mmtVecBdyFrm/1
  mmtArmBdyFrm/1 -> Reshape1/1
  Multiply/1 -> Cross Product/2
  inrt2BdyFrm/1 -> Multiply/1
  forceInrtFrm/1 -> Reshape/1
